simulink model "FMC_AutoTest_Model"  (R2025a)
settings: Solver=daessc  StartTime=0.0  StopTime=stopTime  RelTol=1e-3
settings Model: SimulationMode=accelerator  Creator=mu22504  LastModifiedBy=MW
settings DataIOCC: InspectSignalLogs=on
settings SimscapeCC: SimscapeLogType=all  SimscapeLogSimulationStatistics=on  SimscapeLogToSDI=on

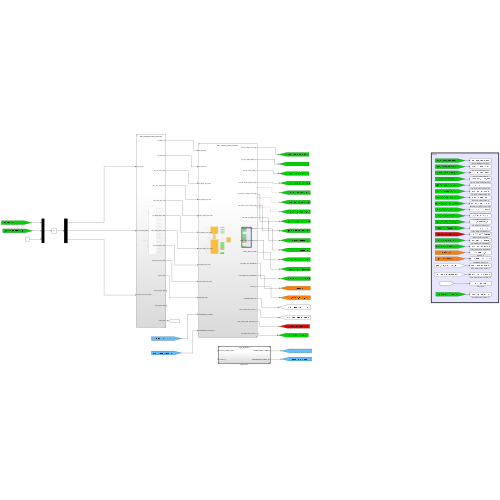
[thumbnail: Simulink's stored preview of the top-level diagram]
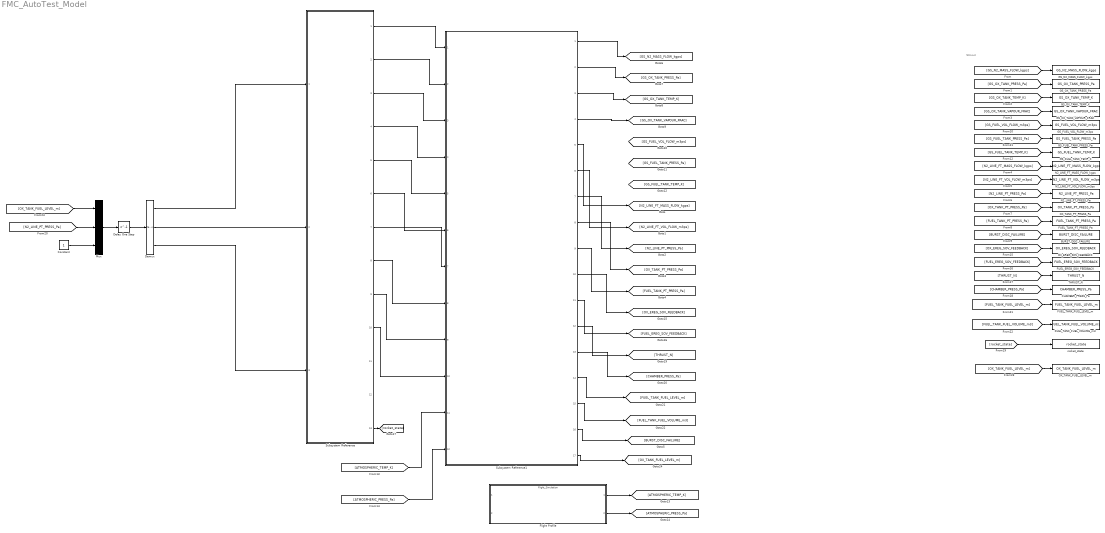
== system FMC_AutoTest_Model ==
  note: SImout
  BURST_DISC_FAILURE : ToWorkspace  VariableName=BURST_DISC_FAILURE  SaveFormat=Timeseries  SampleTime=-1
  CHAMBER_PRESS_Pa : ToWorkspace  VariableName=CHAMBER_PRESS_Pa  SaveFormat=Timeseries  SampleTime=-1
  Constant : Constant
  Delay One Step : Delay  DelayLength=1
  Demux : Demux  Outputs=3
  FUEL_EREG_SOV_FEEDBACK : ToWorkspace  VariableName=FUEL_EREG_SOV_FEEDBACK  SaveFormat=Timeseries  SampleTime=-1
  FUEL_TANK_FUEL_LEVEL_m : ToWorkspace  VariableName=FUEL_TANK_FUEL_LEVEL_m  SaveFormat=Timeseries  SampleTime=-1
  FUEL_TANK_FUEL_VOLUME_m3 : ToWorkspace  VariableName=FUEL_TANK_FUEL_VOLUME_m3  SaveFormat=Timeseries  SampleTime=-1
  FUEL_TANK_PT_PRESS_Pa : ToWorkspace  VariableName=FUEL_TANK_PT_PRESS_Pa  SaveFormat=Timeseries  SampleTime=-1
  "Flight Profile " : ModelReference  ModelNameDialog=Flight_Simulation.slx  SimulationMode=Normal  ModelReferenceVersion=1.3
  GS_FUEL_TANK_PRESS_Pa : ToWorkspace  VariableName=GS_FUEL_TANK_PRESS_Pa  SaveFormat=Timeseries  SampleTime=-1
  GS_FUEL_TANK_TEMP_K : ToWorkspace  VariableName=GS_FUEL_TANK_TEMP_K  SaveFormat=Timeseries  SampleTime=-1
  GS_FUEL_VOL_FLOW_m3ps : ToWorkspace  VariableName=GS_FUEL_VOL_FLOW_m3ps  SaveFormat=Timeseries  SampleTime=-1
  GS_N2_MASS_FLOW_kgps : ToWorkspace  VariableName=GS_N2_MASS_FLOW_kgps  SaveFormat=Timeseries  SampleTime=-1
  GS_OX_TANK_PRESS_Pa : ToWorkspace  VariableName=GS_OX_TANK_PRESS_Pa  SaveFormat=Timeseries  SampleTime=-1
  GS_OX_TANK_TEMP_K : ToWorkspace  VariableName=GS_OX_TANK_TEMP_K  SaveFormat=Timeseries  SampleTime=-1
  GS_OX_TANK_VAPOUR_FRAC : ToWorkspace  VariableName=GS_OX_TANK_VAPOUR_FRAC  SaveFormat=Timeseries  SampleTime=-1
  Mux : Mux  Inputs=3
  N2_LINE_FT_MASS_FLOW_kgps : ToWorkspace  VariableName=N2_LINE_FT_MASS_FLOW_kgps  SaveFormat=Timeseries  SampleTime=-1
  N2_LINE_FT_VOL_FLOW_m3ps : ToWorkspace  VariableName=N2_LINE_FT_VOL_FLOW_m3ps  SaveFormat=Timeseries  SampleTime=-1
  N2_LINE_PT_PRESS_Pa : ToWorkspace  VariableName=N2_LINE_PT_PRESS_Pa  SaveFormat=Timeseries  SampleTime=-1
  OX_EREG_SOV_FEEDBACK : ToWorkspace  VariableName=OX_EREG_SOV_FEEDBACK  SaveFormat=Timeseries  SampleTime=-1
  OX_TANK_FUEL_LEVEL_m : ToWorkspace  VariableName=OX_TANK_FUEL_LEVEL_m  SaveFormat=Timeseries  SampleTime=-1
  OX_TANK_PT_PRESS_Pa : ToWorkspace  VariableName=OX_TANK_PT_PRESS_Pa  SaveFormat=Timeseries  SampleTime=-1
  Subsystem Reference : Subsystem  ReferencedSubsystem=FMC_StateMachineNew_Subsystem
  Subsystem Reference1 : Subsystem  ReferencedSubsystem=FMC_TopLevel_Fluids_Subsystem
  THRUST_N : ToWorkspace  VariableName=THRUST_N  SaveFormat=Timeseries  SampleTime=-1
  rocket_state : ToWorkspace  VariableName=rocket_state  SaveFormat=Timeseries  SampleTime=-1
  wires:
  Subsystem Reference1/5 -> [N2_LINE_FT_MASS_FLOW_kgps]
  Subsystem Reference1/6 -> [N2_LINE_FT_VOL_FLOW_m3ps]
  Subsystem Reference1/7 -> [N2_LINE_PT_PRESS_Pa]
  Subsystem Reference1/8 -> [OX_TANK_PT_PRESS_Pa]
  Subsystem Reference1/9 -> [FUEL_TANK_PT_PRESS_Pa]
  Subsystem Reference1/16 -> [BURST_DISC_FAILURE]
  Subsystem Reference1/1 -> [GS_N2_MASS_FLOW_kgps]
  Subsystem Reference1/2 -> [GS_OX_TANK_PRESS_Pa]
  Subsystem Reference1/3 -> [GS_OX_TANK_TEMP_K]
  Subsystem Reference1/4 -> [GS_OX_TANK_VAPOUR_FRAC]
  [GS_N2_MASS_FLOW_kgps] -> GS_N2_MASS_FLOW_kgps/1
  [GS_OX_TANK_PRESS_Pa] -> GS_OX_TANK_PRESS_Pa/1
  [GS_OX_TANK_TEMP_K] -> GS_OX_TANK_TEMP_K/1
  [GS_OX_TANK_VAPOUR_FRAC] -> GS_OX_TANK_VAPOUR_FRAC/1
  [N2_LINE_FT_MASS_FLOW_kgps] -> N2_LINE_FT_MASS_FLOW_kgps/1
  [BURST_DISC_FAILURE] -> BURST_DISC_FAILURE/1
  [FUEL_TANK_PT_PRESS_Pa] -> FUEL_TANK_PT_PRESS_Pa/1
  [OX_TANK_PT_PRESS_Pa] -> OX_TANK_PT_PRESS_Pa/1
  [N2_LINE_PT_PRESS_Pa] -> N2_LINE_PT_PRESS_Pa/1
  [N2_LINE_FT_VOL_FLOW_m3ps] -> N2_LINE_FT_VOL_FLOW_m3ps/1
  ? -> [GS_FUEL_VOL_FLOW_m3ps]
  ? -> [GS_FUEL_TANK_PRESS_Pa]
  ? -> [GS_FUEL_TANK_TEMP_K]
  [GS_FUEL_VOL_FLOW_m3ps] -> GS_FUEL_VOL_FLOW_m3ps/1
  [GS_FUEL_TANK_PRESS_Pa] -> GS_FUEL_TANK_PRESS_Pa/1
  [GS_FUEL_TANK_TEMP_K] -> GS_FUEL_TANK_TEMP_K/1
  "Flight Profile "/1 -> [ATMOSPHERIC_TEMP_K]
  "Flight Profile "/2 -> [ATMOSPHERIC_PRESS_Pa]
  Subsystem Reference1/10 -> [OX_EREG_SOV_FEEDBACK]
  Subsystem Reference1/11 -> [FUEL_EREG_SOV_FEEDBACK]
  [OX_EREG_SOV_FEEDBACK] -> OX_EREG_SOV_FEEDBACK/1
  [FUEL_EREG_SOV_FEEDBACK] -> FUEL_EREG_SOV_FEEDBACK/1
  Subsystem Reference1/12 -> [THRUST_N]
  Subsystem Reference1/13 -> [CHAMBER_PRESS_Pa]
  [THRUST_N] -> THRUST_N/1
  [CHAMBER_PRESS_Pa] -> CHAMBER_PRESS_Pa/1
  Subsystem Reference1/15 -> [FUEL_TANK_FUEL_VOLUME_m3]
  Subsystem Reference1/14 -> [FUEL_TANK_FUEL_LEVEL_m]
  [FUEL_TANK_FUEL_VOLUME_m3] -> FUEL_TANK_FUEL_VOLUME_m3/1
  [FUEL_TANK_FUEL_LEVEL_m] -> FUEL_TANK_FUEL_LEVEL_m/1
  [ATMOSPHERIC_TEMP_K] -> Subsystem Reference1/11
  [ATMOSPHERIC_PRESS_Pa] -> Subsystem Reference1/12
  Subsystem Reference/1 -> Subsystem Reference1/1
  Subsystem Reference/2 -> Subsystem Reference1/2
  Subsystem Reference/3 -> Subsystem Reference1/3
  Subsystem Reference/4 -> Subsystem Reference1/4
  Subsystem Reference/5 -> Subsystem Reference1/5
  Subsystem Reference/6 -> Subsystem Reference1/6
  Subsystem Reference/7 -> Subsystem Reference1/7
  Subsystem Reference/10 -> Subsystem Reference1/10
  Subsystem Reference/8 -> Subsystem Reference1/8
  Subsystem Reference/9 -> Subsystem Reference1/9
  Subsystem Reference/13 -> [rocket_state]
  [rocket_state] -> rocket_state/1
  Mux/1 -> Delay One Step/1
  Delay One Step/1 -> Demux/1
  Demux/3 -> Subsystem Reference/3
  Demux/2 -> Subsystem Reference/2
  Demux/1 -> Subsystem Reference/1
  Constant/1 -> Mux/3
  [N2_LINE_PT_PRESS_Pa] -> Mux/2
  Subsystem Reference1/17 -> [OX_TANK_FUEL_LEVEL_m]
  [OX_TANK_FUEL_LEVEL_m] -> OX_TANK_FUEL_LEVEL_m/1
  [OX_TANK_FUEL_LEVEL_m] -> Mux/1
